simulink model "convetional_buck"  (R2017b)
settings: Solver=FixedStepAuto  StartTime=0.0  StopTime=1e-3  FixedStep=10e-9  RelTol=1e-3
PostLoadFcn:
  | , if any(exist('dsrtsu_mdlpostloadfcn', 'file') == [2, 3, 6]), try dsrtsu_mdlpostloadfcn('Execute', bdroot); catch fprintf('Error in PostLoadFcn (dsrtsu_mdlpostloadfcn) for model "%s":\n %s\n', bdroot, lasterr); end, end,
values from neighbouring files (symbols this model uses):
  C = 100e-6    (= 0.0001)    [init_conventional_buck.m]
  i_L_init = 1    [init_conventional_buck.m]
  L = 1e-6    (= 1e-06)    [init_conventional_buck.m]
  R = 1    [init_conventional_buck.m]
  r_C = 0*5e-3    (= 0)    [init_conventional_buck.m]
  r_d = 10e-3    (= 0.01)    [init_conventional_buck.m]
  r_L = 10e-3    (= 0.01)    [init_conventional_buck.m]
  rds_on_sw1 = 5e-3    (= 0.005)    [init_conventional_buck.m]
  v_C_init = 3.6    [init_conventional_buck.m]
  Vd = 0.7    [init_conventional_buck.m]
Description:
  | Standard RTI1005 template.
  | Supported MATLAB version:  R2017b.
settings Model: Tag=RTI1005  DSRTSU_INTERNAL_RTI_VER=540  DSRTSU_INTERNAL_RTI_TYPE=rti1005  RTICANMMDATA=struct('GeneralSetupData',struct('modelroot','C:\Projects\Simulink\PE_1\w3','generalsettings',struct('filesettings',struct('destfolder',struct('Name','RTICANMM_FILES','Check',1),'buildfolder',struct('Name','.','Check',1),'AbsDestfolder',struct('Name','C:\Projects\Simulink\PE_1\w3\RTICANMM_FILES'),'AbsBuildfolder',struct('Name','C:\Projects\Simulink\PE_1\w3'))),'options',struct('addpaths',1,'rmpaths',1,'addtrcexclusion',logical(1),'cannavigator',struct('checkmonitoring',0),'show_usrtrc',0,'use_usrtrc',0),'advanced',struct('options',ones(1,100)),'MPSetup',{{}},'RTI',struct('Type','RTI1005','Ver','7.12','Date','02-May-2019'),'modelname','convetional_buck','block','convetional_buck'))  DSRTSU_INTERNAL_RTIFPGA=130  Creator=CA72672  LastModifiedBy=CA72672
settings OptimizationCC: BlockReduction=off  OptimizeBlockIOStorage=off  BufferReuse=off  GlobalBufferReuse=off  ExpressionFolding=off  LocalBlockOutputs=off
settings HardwareCC: ProdBitPerPointer=32  ProdBitPerSizeT=32  ProdBitPerPtrDiffT=32  ProdLargestAtomicInteger=Integer  ProdEndianess=BigEndian  ProdWordSize=32  ProdHWDeviceType=Custom Processor->Custom  TargetIntDivRoundTo=Zero  TargetEndianess=BigEndian  TargetHWDeviceType=Custom Processor->Custom
settings SFSimCC: MATLABDynamicMemAlloc=off
settings RTWCC: SystemTargetFile=rti1005.tlc  MakeCommand=make_rti  TemplateMakefile=rti1005.tmf  Description=dSPACE DS1005 Hardware Platform
settings CodeAppCC: StateflowObjectComments=on
settings STFCustomTargetCC: ParMdlRefBuildCompliant=on  MatFileLogging=on  GRTInterface=off  SystemTargetFile=rti1005.tlc
settings GRTTargetCC: TargetLangStandard=C89/C90 (ANSI)  CompOptLevelCompliant=off  ConcurrentExecutionCompliant=off  CombineOutputUpdateFcns=off  CPPClassGenCompliant=off  UseToolchainInfoCompliant=off
settings ConfigComp: CovMetricSettings=dswe

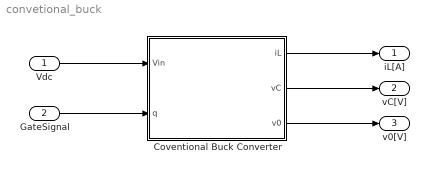
== system convetional_buck ==
  Vdc : Inport
  GateSignal : Inport  Port=2
  Coventional Buck Converter : Subsystem
  iL[A] : Outport
  vC[V] : Outport  Port=2
  v0[V] : Outport  Port=3
  wires:
  Vdc/1 -> Coventional Buck Converter/1(Vin)
  GateSignal/1 -> Coventional Buck Converter/2(q)
  Coventional Buck Converter/1(iL) -> iL[A]/1
  Coventional Buck Converter/2(vC) -> vC[V]/1
  Coventional Buck Converter/3(v0) -> v0[V]/1

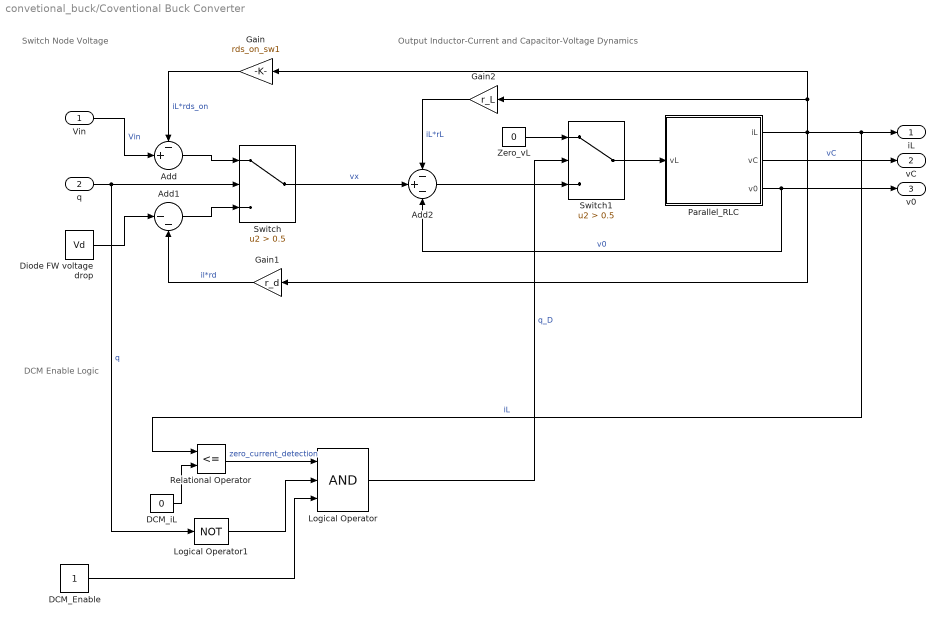
== system convetional_buck/Coventional Buck Converter ==
  note: DCM Enable Logic
  note: Output Inductor-Current and
      | Capacitor-Voltage Dynamics
  note: Switch Node Voltage
  Vin : Inport
  q : Inport  Port=2
  Add : Sum  Inputs=-+|
  Add1 : Sum  Inputs=|--
  Add2 : Sum  Inputs=-+-
  DCM_Enable : Constant
  DCM_iL : Constant  Value=0
  Diode FW voltage drop : Constant  Value=Vd
  Gain : Gain  Gain=rds_on_sw1
  Gain1 : Gain  Gain=r_d
  Gain2 : Gain  Gain=r_L
  Logical Operator : Logic  Inputs=3  IconShape=distinctive  AllPortsSameDT=off  OutDataTypeStr=boolean
  Logical Operator1 : Logic  Operator=NOT  Inputs=3  IconShape=distinctive  AllPortsSameDT=off  OutDataTypeStr=boolean
  Parallel_RLC : Subsystem
  Relational Operator : RelationalOperator  Operator=<=  OutDataTypeStr=boolean  RndMeth=Simplest
  Switch : Switch  Criteria=u2 > Threshold  Threshold=0.5
  Switch1 : Switch  Criteria=u2 > Threshold  Threshold=0.5
  Zero_vL : Constant  Value=0
  iL : Outport
  vC : Outport  Port=2
  v0 : Outport  Port=3
  wires:
  q/1 -> Switch/2, Logical Operator1/1  "q"
  Vin/1 -> Add/2  "Vin"
  Parallel_RLC/3(v0) -> Add2/3, v0/1  "v0"
  Add/1 -> Switch/1
  Parallel_RLC/1(iL) -> Gain1/1, Relational Operator/1, iL/1, Gain/1, Gain2/1  "iL"
  Parallel_RLC/2(vC) -> vC/1  "vC"
  Gain/1 -> Add/1  "iL*rds_on"
  Gain1/1 -> Add1/2  "il*rd"
  Switch/1 -> Add2/2  "vx"
  Add1/1 -> Switch/3
  Diode FW voltage drop/1 -> Add1/1
  Gain2/1 -> Add2/1  "iL*rL"
  Add2/1 -> Switch1/3
  Switch1/1 -> Parallel_RLC/1(vL)
  Logical Operator/1 -> Switch1/2  "q_D"
  Zero_vL/1 -> Switch1/1
  DCM_iL/1 -> Relational Operator/2
  Relational Operator/1 -> Logical Operator/1  "zero_current_detection"
  Logical Operator1/1 -> Logical Operator/2
  DCM_Enable/1 -> Logical Operator/3

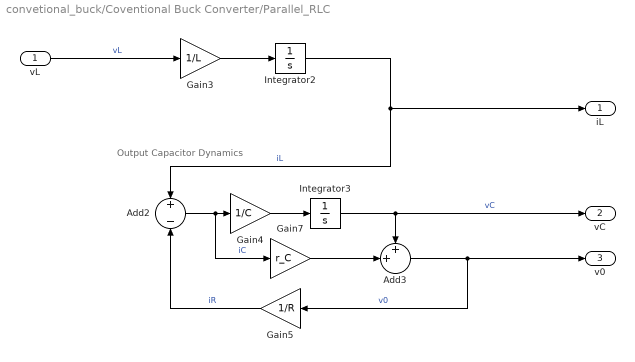
== system convetional_buck/Coventional Buck Converter/Parallel_RLC ==
  note: Output Capacitor Dynamics
  vL : Inport
  Add2 : Sum  Inputs=+|-
  Add3 : Sum  Inputs=++|
  Gain3 : Gain  Gain=1/L
  Gain4 : Gain  Gain=1/C
  Gain5 : Gain  Gain=1/R
  Gain7 : Gain  Gain=r_C
  Integrator2 : Integrator  InitialCondition=i_L_init
  Integrator3 : Integrator  InitialCondition=v_C_init
  iL : Outport
  vC : Outport  Port=2
  v0 : Outport  Port=3
  wires:
  vL/1 -> Gain3/1  "vL"
  Gain3/1 -> Integrator2/1
  Integrator2/1 -> Add2/1, iL/1  "iL"
  Gain4/1 -> Integrator3/1
  Add2/1 -> Gain7/1, Gain4/1  "iC"
  Gain5/1 -> Add2/2  "iR"
  Integrator3/1 -> vC/1, Add3/1  "vC"
  Gain7/1 -> Add3/2
  Add3/1 -> v0/1, Gain5/1  "v0"
